simulink model "MainLV1"  (R2024a)
settings: Solver=FixedStepDiscrete  StartTime=0.0  StopTime=Inf  RelTol=1e-3  EnableMultiTasking=on
PreLoadFcn:
  | RTWConfigurationCB('preloadfcn', bdroot);
model workspace (MAT data in the model file):
  fault_count = 0
libraries: canmsglib x11, c280xlib x11, c2837xDlib x5, c2802xlib x5, simulink x4, slpidlib x1
settings Model: ExtModeTrigDuration=8  Creator=Brian  LastModifiedBy=benjaminlevin
settings SolverCC: AutoInsertRateTranBlk=on
settings OptimizationCC: DefaultUnderspecifiedDataType=single  EnhancedBackFolding=on  PassReuseOutputArgsAs=Individual arguments  MaxStackSize=1024  OptimizeBlockOrder=speed  DifferentSizesBufferReuse=on  OptimizationCustomize=off  DenormalBehavior=FlushToZero  EfficientTunableParamExpr=on
settings DebuggingCC: ParameterTunabilityLossMsg=error
settings HardwareCC: ProdBitPerChar=16  ProdBitPerInt=16  ProdBitPerPointer=32  ProdBitPerSizeT=32  ProdBitPerPtrDiffT=32  ProdLargestAtomicInteger=Integer  ProdLargestAtomicFloat=None  ProdWordSize=16  ProdLongLongMode=on  ProdHWDeviceType=Texas Instruments->C2000  HardwareBoardFeatureSet=SoCBlockset
settings ModelReferenceCC: EnableRefExpFcnMdlSchedulingChecks=on  ModelReferenceNumInstancesAllowed=Single
settings SFSimCC: MATLABDynamicMemAlloc=off
settings RTWCC: Description=Embedded Coder  SystemTargetFile=ert.tlc  HardwareBoard=TI Delfino F28379D LaunchPad  TemplateMakefile=ert_default_tmf  Toolchain=Texas Instruments Code Composer Studio (C2000)  CodeProfilingSaveOptions=MetricsOnly  GPUComputeCapability=3.5
settings CodeAppCC: ForceParamTrailComments=on  IgnoreCustomStorageClasses=off  OperatorAnnotations=on  SimulinkDataObjDesc=on  SFDataObjDesc=on  InsertBlockDesc=on
settings ERTTargetCC: CodeReplacementLibrary=TI C28x  ExtModeTransport=4  ExtModeStaticAlloc=on  ExtModeAutomaticAllocSize=off  ExtModeStaticAllocSize=10000  ExtModeMexFile=ext_xcp  ExtModeIntrfLevel=Level2 - Open

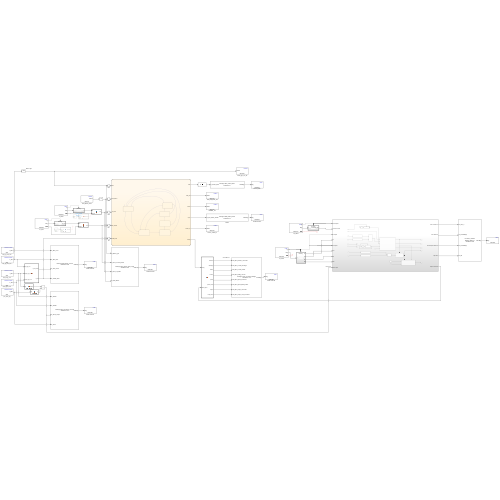
[thumbnail: Simulink's stored preview of the top-level diagram]
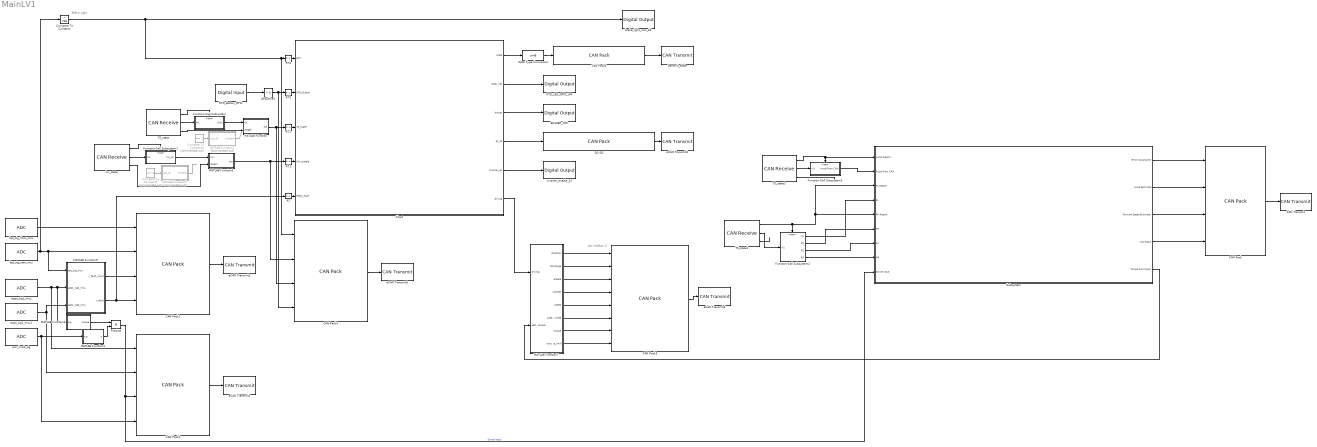
== system MainLV1 ==
  note: Brake Light
  note: can mailbox 3
  BUZZER_105 : c2837xDlib/Digital Output  GPIO_Number=GPIO104~GPIO111  GPIO_Bit0=off  GPIO_BIT0_Toggle=off  GPIO_Bit1=on  GPIO_BIT1_Toggle=off  GPIO_Bit2=off  GPIO_BIT2_Toggle=off  GPIO_Bit3=off  GPIO_BIT3_Toggle=off  GPIO_Bit4=off  GPIO_BIT4_Toggle=off  GPIO_Bit5=off  GPIO_BIT5_Toggle=off  GPIO_Bit6=off  GPIO_BIT6_Toggle=off  GPIO_Bit7=off  GPIO_BIT7_Toggle=off
  CAN Pack : canmsglib/CAN Pack  MsgList=(none)  MsgName=M404_LV  MsgIDType=Standard (11-bit identifier)  MsgIdentifier=404  MsgLength=8  Remote=off  ApplyMinMax=off  BusOutput=off  SignalInfo={ 'LV_COV_V', '32', '8', 'LE', 'unsigned', 'Standard', '0', '0.02', '0', '0', '5.1'; 'LV_FILTERED_A', '16', '16', 'LE', 'unsigned', 'Standard', '0', '5e-05', '0', '0', '3.2767'; 'LV_FILTERED_V', '0', '16', 'LE', 'unsigned', 'Standard', '0', '0.0025', '0', '0', '163.8375'; 'LV_SR', '48', '16', 'LE', 'signed', 'Standard', '0', '0.0001', '0', '-3.2768', '3.2767' }
      settings: LibrarySourceBlock=c2000lib/Target Communication/CAN Pack  DataFormat=manually specified signals
  CAN Pack1 : canmsglib/CAN Pack  MsgList=(none)  MsgName=M402_Brake_Controls  MsgIDType=Standard (11-bit identifier)  MsgIdentifier=402  MsgLength=6  Remote=off  ApplyMinMax=off  BusOutput=off  SignalInfo={'LV_BPT_Front','16','16','LE','unsigned','Standard','0','1','0','-Inf','Inf';'LV_BPT_Rear','0','16','LE','unsigned','Standard','0','1','0','-Inf','Inf';'LV_Fault_Count','40','8','LE','unsigned','Standard','0','1','0','-Inf','Inf';'LV_Pedals_Fault','32','8','LE','signed','Standard','0','1','0','-Inf','Inf'}
      settings: DataFormat=manually specified signals
  CAN Pack2 : canmsglib/CAN Pack  MsgList=(none)  MsgName=M401_Accelerator_Controls  MsgIDType=Standard (11-bit identifier)  MsgIdentifier=401  MsgLength=8  Remote=off  ApplyMinMax=off  BusOutput=off  SignalInfo={'LV_APPS1','0','16','LE','unsigned','Standard','0','1','0','-Inf','Inf';'LV_APPS2','16','16','LE','unsigned','Standard','0','1','0','-Inf','Inf';'LV_Driver_Torque','48','16','LE','signed','Standard','0','0.1','0','-3276.8','3276.7';'LV_Knob','32','16','LE','unsigned','Standard','0','1','0','-Inf','Inf'}
      settings: DataFormat=manually specified signals
  CAN Pack3 : canmsglib/CAN Pack  MsgList=(none)  MsgName=M176_Command_Message  MsgIDType=Standard (11-bit identifier)  MsgIdentifier=176  MsgLength=8  Remote=off  ApplyMinMax=off  BusOutput=off  SignalInfo={'VCU_INV_Direction_Command','32','1','LE','unsigned','Standard','0','1','0','0','1';'VCU_INV_Inverter_Discharge','41','1','LE','unsigned','Standard','0','1','0','0','1';'VCU_INV_Inverter_Enable','40','1','LE','unsigned','Standard','0','1','0','0','1';'VCU_INV_Rolling_Counter','44','4','LE','unsigned','Standard','0','1','0','0','15';'VCU_INV_Speed_Command','16','16','LE','signed','Standard','0','1','0','-32768','32767';'VCU_INV_Speed_Mode_Enable','42','1','LE','unsigned','Standard','0','1','0','0','1';'VCU_INV_Torque_Command','0','16','LE','signed','Standard','0','0.1','0','-3276.8','3276.7';'VCU_INV_Torque_Limit_Command','48','16','LE','signed','Standard','0','0.1','0','-3276.8','3276.7'}
      settings: DataFormat=manually specified signals
  CAN Pack4 : canmsglib/CAN Pack  MsgList=(none)  MsgName=M001_Vehicle_State  MsgIDType=Standard (11-bit identifier)  MsgIdentifier=1  MsgLength=1  Remote=off  ApplyMinMax=off  BusOutput=off  SignalInfo={'LV_Vehicle_State','0','8','LE','signed','Standard','0','1','0','-Inf','Inf'}
      settings: DataFormat=manually specified signals
  CAN Pack5 : canmsglib/CAN Pack  MsgList=(none)  MsgName=M403_Vehicle_State_Inputs  MsgIDType=Standard (11-bit identifier)  MsgIdentifier=403  MsgLength=4  Remote=off  ApplyMinMax=off  BusOutput=off  SignalInfo={'LV_Brake_Light','0','8','LE','unsigned','Standard','0','1','0','-Inf','Inf';'LV_Echo_Inverter_Enable','8','8','LE','signed','Standard','0','1','0','-Inf','Inf';'LV_Echo_TS_State','16','8','LE','signed','Standard','0','1','0','-Inf','Inf';'LV_RTD_Button','24','8','LE','unsigned','Standard','0','1','0','-Inf','Inf'}
      settings: DataFormat=manually specified signals
  CAN Transmit : c280xlib/CAN Transmit  chipFamily=C280x  useModule=CAN_A  mailboxNo=11  messageID=404  messageType=Standard (11-bit identifier)  enableBlockingMode=off  postInterrupt=off  interruptLine=0
  Chart : Stateflow chart  TreatAsAtomicUnit=on  SystemSampleTime=0.01
      settings: RTWSystemCode=Inline  RTWFcnNameOpts=Use subsystem name  RTWFileNameOpts=Use subsystem name  PortSchema="{\"entries\":[{\"content\":{\"sides\":[{\"content\":{\"connectorIds\":[\"In1\",\"In2\",\"In5\",\"In4\",\"In3\"]},\"type\":\"ConnectorPlacement.EquallySpacedRectSide\",\"uuid\":\"e489c846-491e-4e82-9c5f-b669d7c96954\"},{\"content\":{\"connectorIds\":[\"Out1\",\"Out2\",\"Out3\",\"Out4\",\"Out5\",\"Out6\"],\"side\":\"RIGHT\"},\"type\":\"ConnectorPlacement.EquallySpacedRectSide\",\"uuid\":\"cbb46da5-6eb6-44f9-baf3-a24ec6c96225\"},{\"content\":{\"side\":\"TOP\"},\"type\":\"ConnectorPlacement.EquallySpacedRectSide\",\"uuid\":\"c6202e3b-aafb-4b81-a309-4cc98c9bb853\"},{\"content\":{\"side\":\"BOTTOM\"},\"type\":\"ConnectorPlacement.EquallySpacedRectSide\",\"uuid\":\"d6a20d7c-ea9b-4afd-8884-952a45f498ea\"}]},\"type\":\"ConnectorPlacement.EquallySpacedConnector\",\"uuid\":\"7c3bea70-19b9-40c4-b7cb-79b1c3f0d3c0\"}],\"packageUris\":[\"http://schema.mathworks.com/mf0/Connector/R2020b\"],\"version\":\"1.0\"}"
  Compare To Constant : simulink/Logic and Bit Operations/Compare To Constant  relop=>  const=728  OutDataTypeStr=boolean
  Compare To Constant4 : simulink/Logic and Bit Operations/Compare To Constant  Commented=on  relop===  const=1  OutDataTypeStr=boolean
  Compare To Constant5 : simulink/Logic and Bit Operations/Compare To Constant  Commented=on  relop===  const=8  OutDataTypeStr=boolean
  DC-DC : canmsglib/CAN Pack  MsgList=(none)  MsgName=M003_DCDC_Enable  MsgIDType=Standard (11-bit identifier)  MsgIdentifier=3  MsgLength=1  Remote=off  ApplyMinMax=off  BusOutput=off  SignalInfo={'LV_ACC_DCDC_Enable','0','8','LE','signed','Standard','0','1','0','-Inf','Inf'}
      settings: DataFormat=manually specified signals
  Data Type Conversion : DataTypeConversion  OutDataTypeStr=uint8  SaturateOnIntegerOverflow=off  RndMeth=Floor
  Function-Call Subsystem : Subsystem  TreatAsAtomicUnit=on
  Function-Call Subsystem1 : Subsystem  TreatAsAtomicUnit=on
  Function-Call Subsystem2 : Subsystem  TreatAsAtomicUnit=on
  Function-Call Subsystem3 : Subsystem  TreatAsAtomicUnit=on
  IsPositive3 : simulink/Logic and Bit Operations/Compare To Zero  relop=>  OutDataTypeStr=boolean
  MATLAB Function : MATLAB Function  TreatAsAtomicUnit=on
  MATLAB Function1 : MATLAB Function  TreatAsAtomicUnit=on
  MATLAB Function2 : MATLAB Function  Commented=on  TreatAsAtomicUnit=on
  MATLAB Function3 : MATLAB Function  TreatAsAtomicUnit=on
  MATLAB Function4 : MATLAB Function  TreatAsAtomicUnit=on
  MATLAB Function5 : MATLAB Function  Commented=on  TreatAsAtomicUnit=on
  MATLAB Function7 : MATLAB Function  TreatAsAtomicUnit=on
  MATLAB Function9 : MATLAB Function  TreatAsAtomicUnit=on
  Product : Product  OutDataTypeStr=double
  RT{,1..4} (5 alike) : RateTransition  OutPortSampleTime=0.01
  RTD_Button_GPIO : c2837xDlib/Digital Input  GPIO_Number=GPIO32~GPIO39  GPIO_Bit0=on  GPIO_Bit1=off  GPIO_Bit2=off  GPIO_Bit3=off  GPIO_Bit4=off  GPIO_Bit5=off  GPIO_Bit6=off  GPIO_Bit7=off  sampleTime=0.1  dataType=uint8  GPIO_Bit0_Qualification=Sync to SYSCLKOUT  GPIO_Bit1_Qualification=Sync to SYSCLKOUT  GPIO_Bit2_Qualification=Sync to SYSCLKOUT  GPIO_Bit3_Qualification=Sync to SYSCLKOUT  GPIO_Bit4_Qualification=Sync to SYSCLKOUT  GPIO_Bit5_Qualification=Sync to SYSCLKOUT  GPIO_Bit6_Qualification=Sync to SYSCLKOUT  GPIO_Bit7_Qualification=Sync to SYSCLKOUT  Qualification_Period=-1
  RTD_LED_GPIO_104 : c2837xDlib/Digital Output  GPIO_Number=GPIO104~GPIO111  GPIO_Bit0=on  GPIO_BIT0_Toggle=off  GPIO_Bit1=off  GPIO_BIT1_Toggle=off  GPIO_Bit2=off  GPIO_BIT2_Toggle=off  GPIO_Bit3=off  GPIO_BIT3_Toggle=off  GPIO_Bit4=off  GPIO_BIT4_Toggle=off  GPIO_Bit5=off  GPIO_BIT5_Toggle=off  GPIO_Bit6=off  GPIO_BIT6_Toggle=off  GPIO_Bit7=off  GPIO_BIT7_Toggle=off
  Subsystem : Subsystem
  TS_state : c280xlib/CAN Receive  chipFamily=C280x  useModule=CAN_B  mailboxNo=2  messageID=2  messageType=Standard (11-bit identifier)  enableAcceptanceFiltering=off  messageIDMask=0  sampleTime=.25  dataType=CAN_MESSAGE_TYPE  outputAction=Reset all fields to zero  initValue=0  outputMessageID=off  outputMessageLength=on  outputMessageTimeStamp=off  postInterrupt=off  interruptLine=0
  TS_state1 : c280xlib/CAN Receive  chipFamily=C280x  useModule=CAN_B  mailboxNo=9  messageID=51  messageType=Standard (11-bit identifier)  enableAcceptanceFiltering=off  messageIDMask=0  sampleTime=-1  dataType=CAN_MESSAGE_TYPE  outputAction=Reset all fields to zero  initValue=0  outputMessageID=off  outputMessageLength=on  outputMessageTimeStamp=off  postInterrupt=on  interruptLine=0
  TS_state2 : c280xlib/CAN Receive  chipFamily=C280x  useModule=CAN_B  mailboxNo=10  messageID=52  messageType=Standard (11-bit identifier)  enableAcceptanceFiltering=off  messageIDMask=0  sampleTime=-1  dataType=CAN_MESSAGE_TYPE  outputAction=Reset all fields to zero  initValue=0  outputMessageID=off  outputMessageLength=on  outputMessageTimeStamp=off  postInterrupt=on  interruptLine=0
  apps_sig1_mcu : c2802xlib/ADC  blkParamProc=C2000_Type4  ADCModule=A  samplingMode=Single sample mode  ADCResolution=12-bit (Single-ended input)  useSOC1=SOC15  useSOC2=SOC0_SOC1  SOCAcquisitionWindow=60  SOCTriggerSource=Software  SOCInterruptTrigger=No ADCINT  Ts=0.001  dType=uint16  postInterrupt=off  interruptSel=ADCINT1  ADCINTContinuous=on  endma=off  chdma=1  conv1=ADCINA0  conv2=ADCINA0 and ADCINB0  conv1_Type4=ADCIN3  conv2_Type4=ADCIN0 and ADCIN1
  apps_sig2_mcu1 : c2802xlib/ADC  blkParamProc=C2000_Type4  ADCModule=C  samplingMode=Single sample mode  ADCResolution=12-bit (Single-ended input)  useSOC1=SOC10  useSOC2=SOC0_SOC1  SOCAcquisitionWindow=60  SOCTriggerSource=Software  SOCInterruptTrigger=No ADCINT  Ts=0.001  dType=uint16  postInterrupt=off  interruptSel=ADCINT1  ADCINTContinuous=on  endma=off  chdma=1  conv1=ADCINA0  conv2=ADCINA0 and ADCINB0  conv1_Type4=ADCIN2  conv2_Type4=ADCIN0 and ADCIN1
  bpt_sig_front_mcu : c2802xlib/ADC  blkParamProc=C2000_Type4  ADCModule=B  samplingMode=Single sample mode  ADCResolution=12-bit (Single-ended input)  useSOC1=SOC6  useSOC2=SOC0_SOC1  SOCAcquisitionWindow=60  SOCTriggerSource=Software  SOCInterruptTrigger=No ADCINT  Ts=0.001  dType=uint16  postInterrupt=off  interruptSel=ADCINT1  ADCINTContinuous=on  endma=off  chdma=1  conv1=ADCINA0  conv2=ADCINA0 and ADCINB0  conv1_Type4=ADCIN3  conv2_Type4=ADCIN0 and ADCIN1
  bpt_sig_rear_mcu : c2802xlib/ADC  blkParamProc=C2000_Type4  ADCModule=C  samplingMode=Single sample mode  ADCResolution=12-bit (Single-ended input)  useSOC1=SOC6  useSOC2=SOC0_SOC1  SOCAcquisitionWindow=60  SOCTriggerSource=Software  SOCInterruptTrigger=No ADCINT  Ts=0.001  dType=uint16  postInterrupt=off  interruptSel=ADCINT1  ADCINTContinuous=on  endma=off  chdma=1  conv1=ADCINA0  conv2=ADCINA0 and ADCINB0  conv1_Type4=ADCIN3  conv2_Type4=ADCIN0 and ADCIN1
  brake_light_mcu_60 : c2837xDlib/Digital Output  GPIO_Number=GPIO56~GPIO63  GPIO_Bit0=off  GPIO_BIT0_Toggle=off  GPIO_Bit1=off  GPIO_BIT1_Toggle=off  GPIO_Bit2=off  GPIO_BIT2_Toggle=off  GPIO_Bit3=off  GPIO_BIT3_Toggle=off  GPIO_Bit4=on  GPIO_BIT4_Toggle=off  GPIO_Bit5=off  GPIO_BIT5_Toggle=off  GPIO_Bit6=off  GPIO_BIT6_Toggle=off  GPIO_Bit7=off  GPIO_BIT7_Toggle=off
  eCAN Transmit1 : c280xlib/CAN Transmit  chipFamily=C280x  useModule=CAN_B  mailboxNo=6  messageID=401  messageType=Standard (11-bit identifier)  enableBlockingMode=off  postInterrupt=off  interruptLine=0
  eCAN Transmit2 : c280xlib/CAN Transmit  chipFamily=C280x  useModule=CAN_B  mailboxNo=7  messageID=402  messageType=Standard (11-bit identifier)  enableBlockingMode=off  postInterrupt=off  interruptLine=0
  eCAN Transmit3 : c280xlib/CAN Transmit  chipFamily=C280x  useModule=CAN_B  mailboxNo=3  messageID=3  messageType=Standard (11-bit identifier)  enableBlockingMode=off  postInterrupt=off  interruptLine=0
  eCAN Transmit4 : c280xlib/CAN Transmit  chipFamily=C280x  useModule=CAN_B  mailboxNo=4  messageID=192  messageType=Standard (11-bit identifier)  enableBlockingMode=off  postInterrupt=off  interruptLine=0
  eCAN Transmit5 : c280xlib/CAN Transmit  chipFamily=C280x  useModule=CAN_B  mailboxNo=8  messageID=403  messageType=Standard (11-bit identifier)  enableBlockingMode=off  postInterrupt=off  interruptLine=0
  inv_state : c280xlib/CAN Receive  chipFamily=C280x  useModule=CAN_B  mailboxNo=5  messageID=154  messageType=Standard (11-bit identifier)  enableAcceptanceFiltering=off  messageIDMask=0  sampleTime=.25  dataType=CAN_MESSAGE_TYPE  outputAction=Reset all fields to zero  initValue=0  outputMessageID=off  outputMessageLength=on  outputMessageTimeStamp=off  postInterrupt=off  interruptLine=0
  inverter_enable_22 : c2837xDlib/Digital Output  GPIO_Number=GPIO16~GPIO23  GPIO_Bit0=off  GPIO_BIT0_Toggle=off  GPIO_Bit1=off  GPIO_BIT1_Toggle=off  GPIO_Bit2=off  GPIO_BIT2_Toggle=off  GPIO_Bit3=off  GPIO_BIT3_Toggle=off  GPIO_Bit4=off  GPIO_BIT4_Toggle=off  GPIO_Bit5=off  GPIO_BIT5_Toggle=off  GPIO_Bit6=on  GPIO_BIT6_Toggle=off  GPIO_Bit7=off  GPIO_BIT7_Toggle=off
  pwr_knob_sig : c2802xlib/ADC  blkParamProc=C2000_Type4  ADCModule=B  samplingMode=Single sample mode  ADCResolution=12-bit (Single-ended input)  useSOC1=SOC10  useSOC2=SOC0_SOC1  SOCAcquisitionWindow=60  SOCTriggerSource=Software  SOCInterruptTrigger=No ADCINT  Ts=0.001  dType=uint16  postInterrupt=off  interruptSel=ADCINT1  ADCINTContinuous=on  endma=off  chdma=1  conv1=ADCINA0  conv2=ADCINA0 and ADCINB0  conv1_Type4=ADCIN2  conv2_Type4=ADCIN0 and ADCIN1
  transmit_state : c280xlib/CAN Transmit  chipFamily=C280x  useModule=CAN_B  mailboxNo=1  messageID=1  messageType=Standard (11-bit identifier)  enableBlockingMode=off  postInterrupt=off  interruptLine=0
  wires:
  Data Type Conversion/1 -> CAN Pack4/1
  TS_state/2 -> Function-Call Subsystem/1(In1)
  MATLAB Function9/2(r_fault) -> RT/1, CAN Pack1/4
  Function-Call Subsystem/1(Out1) -> MATLAB Function/1(ts)
  TS_state/1 -> Function-Call Subsystem/Trigger
  CAN Pack4/1 -> transmit_state/1
  bpt_sig_rear_mcu/1 -> CAN Pack1/2, MATLAB Function9/1(bpt_sig_mcu), Compare To Constant/1
  apps_sig1_mcu/1 -> CAN Pack2/1, MATLAB Function4/1(sig), MATLAB Function9/2(apps_sig1_mcu)
  apps_sig2_mcu1/1 -> MATLAB Function9/3(apps_sig2_mcu), CAN Pack2/2
  RTD_Button_GPIO/1 -> IsPositive3/1
  CAN Pack1/1 -> eCAN Transmit2/1
  pwr_knob_sig/1 -> CAN Pack2/4, MATLAB Function1/1(sig)
  MATLAB Function1/1(p) -> Product/2
  MATLAB Function4/1(torque) -> Product/1
  DC-DC/1 -> eCAN Transmit3/1
  Chart/1(state) -> Data Type Conversion/1
  CAN Pack3/1 -> eCAN Transmit4/1
  bpt_sig_front_mcu/1 -> CAN Pack1/1
  MATLAB Function9/1(r_fault_count) -> CAN Pack1/3
  CAN Pack2/1 -> eCAN Transmit1/1
  TS_state/3 -> MATLAB Function/2(length)
  Compare To Constant4/1 -> MATLAB Function2/1(can_ok)
  MATLAB Function2/1(timeout) -> ?
  inv_state/1 -> Function-Call Subsystem1/Trigger
  inv_state/2 -> Function-Call Subsystem1/1(In1)
  inv_state/3 -> MATLAB Function3/2(length)
  Compare To Constant5/1 -> MATLAB Function5/1(can_ok)
  Function-Call Subsystem1/1(inv_en) -> MATLAB Function3/1(inv)
  MATLAB Function5/1(timeout) -> ?
  Chart/3(buzzer) -> BUZZER_105/1
  Chart/4(dc_dc) -> DC-DC/1
  Chart/5(inverter_en) -> inverter_enable_22/1
  Chart/6(driving) -> MATLAB Function7/1(driving)
  MATLAB Function7/1(direction) -> CAN Pack3/1
  MATLAB Function7/2(discharge) -> CAN Pack3/2
  MATLAB Function7/3(enable) -> CAN Pack3/3
  MATLAB Function7/5(speed) -> CAN Pack3/5
  MATLAB Function7/4(counter) -> CAN Pack3/4
  MATLAB Function7/6(speed_mode) -> CAN Pack3/6
  MATLAB Function7/7(torque) -> CAN Pack3/7
  MATLAB Function7/8(torque_limit) -> CAN Pack3/8
  Compare To Constant/1 -> brake_light_mcu_60/1, CAN Pack5/1, RT4/1
  Chart/2(ready_led) -> RTD_LED_GPIO_104/1
  CAN Pack5/1 -> eCAN Transmit5/1
  IsPositive3/1 -> CAN Pack5/4, RT3/1
  MATLAB Function/1(out) -> CAN Pack5/3, RT2/1
  MATLAB Function3/1(out) -> CAN Pack5/2, RT1/1
  RT/1 -> Chart/3(Pedal_Fault)
  RT1/1 -> Chart/4(INV_enable)
  RT2/1 -> Chart/5(TS_state)
  RT3/1 -> Chart/2(RTD_Button)
  RT4/1 -> Chart/1(BPT)
  Product/1 -> Subsystem/9(Driver Input), CAN Pack2/3  "Driver Input"
  Subsystem/5(Torque Command) -> MATLAB Function7/2(pedal_torque)
  TS_state1/1 -> Subsystem/3(FL Report), Subsystem/5(FR Report), Function-Call Subsystem2/Trigger
  TS_state1/2 -> Function-Call Subsystem2/1(In1)
  TS_state1/3 -> ?
  TS_state2/2 -> Function-Call Subsystem3/1(In1)
  TS_state2/3 -> ?
  Subsystem/1(Error Covariance) -> CAN Pack/1
  Subsystem/2(Accel Estimate) -> CAN Pack/2
  Subsystem/3(Forward Speed Estimate) -> CAN Pack/3
  Subsystem/4(Slip Ratio) -> CAN Pack/4
  CAN Pack/1 -> CAN Transmit/1
  TS_state2/1 -> Subsystem/1(Accel Report), Function-Call Subsystem3/Trigger
  Function-Call Subsystem2/1(FL) -> Subsystem/4(FL)
  Function-Call Subsystem2/2(FR) -> Subsystem/6(FR)
  Function-Call Subsystem2/3(RL) -> Subsystem/7(RL)
  Function-Call Subsystem2/4(RR) -> Subsystem/8(RR)
  Function-Call Subsystem3/1(Accel from CAN) -> Subsystem/2(Accel from CAN)

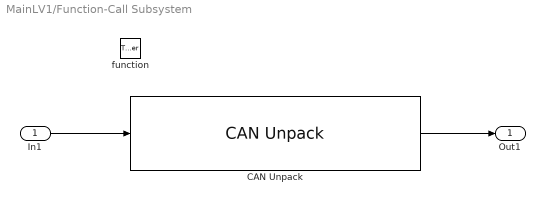
== system MainLV1/Function-Call Subsystem ==
  In1 : Inport
  function : TriggerPort  TriggerType=function-call  VariantControl=(inherit)
  CAN Unpack : canmsglib/CAN Unpack  MsgList=(none)  MsgName=M002_TS_State  MsgIDType=Standard (11-bit identifier)  MsgIdentifier=2  MsgLength=1  SignalInfo={'ACC_TS_State','0','8','LE','signed','Standard','0','1','0','-Inf','Inf'}  IDPort=off  TimestampPort=off  ErrorPort=off  RemotePort=off  LengthPort=off  StatusPort=off  ApplyMinMax=off
  Out1 : Outport  OutDataTypeStr=int8
  wires:
  In1/1 -> CAN Unpack/1
  CAN Unpack/1 -> Out1/1

== system MainLV1/Function-Call Subsystem1 ==
  In1 : Inport
  function : TriggerPort  TriggerType=function-call  VariantControl=(inherit)
  CAN Unpack : canmsglib/CAN Unpack  CANdbFile=C:\Users\lukeh\Documents\FSAE\EV24-Software\CAN\20240129 Gen5 CAN DB.dbc  MsgList=(none)  MsgName=M154_Internal_States  MsgIDType=Standard (11-bit identifier)  MsgIdentifier=154  MsgLength=8  SignalInfo={'INV_BMS_Active','57','1','LE','unsigned','Standard','0','1','0','0','1';'INV_BMS_Torque_Limiting','58','1','LE','unsigned','Standard','0','1','0','0','1';'INV_Burst_Model_Mode','49','1','LE','unsigned','Standard','0','1','0','0','1';'INV_Direction_Command','56','1','LE','unsigned','Standard','0','1','0','0','1';'INV_Inverter_Command_Mode','40','1','LE','unsigned','Standard','0','1','0','0','1';'INV_Inverter_Discharge_State','37','3','LE','unsigned','Standard','0','1','0','0','7';'INV_Inverter_Enable_Lockout','55','1','LE','unsigned','Standard','0','1','0','0','1';'INV_Inverter_Enable_State','48','1','LE','unsigned','Standard','0','1','0','0','1';'INV_Inverter_Run_Mode','32','1','LE','unsigned','Standard','0','1','0','0','1';'INV_Inverter_State','16','8','LE','unsigned','Standard','0','1','0','0','255';'INV_Key_Switch_Start_Status','54','1','LE','unsigned','Standard','0','1','0','0','1';'INV_Limit_Coolant_Derating','62','1','LE','unsigned','Standard','0','1','0','0','1';'INV_Limit_Hot_Spot','60','1','LE','unsigned','Standard','0','1','0','0','1';'INV_Limit_Max_Speed','59','1','LE','unsigned','Standard','0','1','0','0','1';'INV_Limit_Stall_Burst_Model','63','1','LE','unsigned','Standard','0','1','0','0','1';'INV_Low_Speed_Limiting','61','1','LE','unsigned','Standard','0','1','0','0','1';'INV_PWM_Frequency','8','8','LE','unsigned','Standard','0','1','0','0','255';'INV_Relay_1_Status','24','1','LE','unsigned','Standard','0','1','0','0','1';'INV_Relay_2_Status','25','1','LE','unsigned','Standard','0','1','0','0','1';'INV_Relay_3_Status','26','1','LE','unsigned','Standard','0','1','0','0','1';'INV_Relay_4_Status','27','1','LE','unsigned','Standard','0','1','0','0','1';'INV_Relay_5_Status','28','1','LE','unsigned','Standard','0','1','0','0','1';'INV_Relay_6_Status','29','1','LE','unsigned','Standard','0','1','0','0','1';'INV_Rolling_Counter','44','4','LE','unsigned','Standard','0','1','0','0','15';'INV_Self_Sensing_Assist_Enable','33','1','LE','unsigned','Standard','0','1','0','0','1';'INV_VSM_State','0','8','LE','unsigned','Standard','0','1','0','0','15'}  IDPort=off  TimestampPort=off  ErrorPort=off  RemotePort=off  LengthPort=off  StatusPort=off  ApplyMinMax=off
      settings: DataFormat=CANdb specified signals
  inv_en : Outport  OutDataTypeStr=uint8
  wires:
  In1/1 -> CAN Unpack/1
  CAN Unpack/8 -> inv_en/1

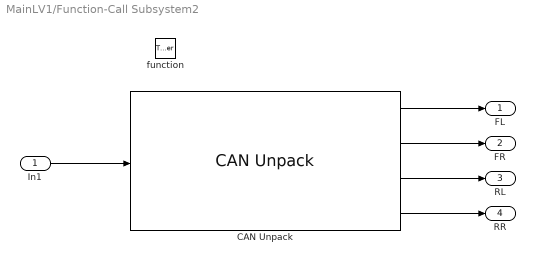
== system MainLV1/Function-Call Subsystem2 ==
  In1 : Inport
  function : TriggerPort  TriggerType=function-call  VariantControl=(inherit)
  CAN Unpack : canmsglib/CAN Unpack  CANdbFile=C:\Users\xudon\OneDrive\Columbia University\FSAE\LV\EV25_CAN.dbc  MsgList=M051_Wheel_Speeds  MsgName=M051_Wheel_Speeds  MsgIDType=Standard (11-bit identifier)  MsgIdentifier=51  MsgLength=8  SignalInfo={ 'SEN_WSS_FL', '0', '16', 'LE', 'unsigned', 'Standard', '0', '0.0025', '0', '0', '163.8375'; 'SEN_WSS_FR', '16', '16', 'LE', 'unsigned', 'Standard', '0', '0.0025', '0', '0', '163.8375'; 'SEN_WSS_RL', '32', '16', 'LE', 'unsigned', 'Standard', '0', '0.0025', '0', '0', '163.8375'; 'SEN_WSS_RR', '48', '16', 'LE', 'unsigned', 'Standard', '0', '0.0025', '0', '0', '163.8375' }  IDPort=off  TimestampPort=off  ErrorPort=off  RemotePort=off  LengthPort=off  StatusPort=off  ApplyMinMax=off
      settings: DataFormat=CANdb specified signals
  FL : Outport  OutDataTypeStr=int8
  FR : Outport  Port=2  OutDataTypeStr=int8
  RL : Outport  Port=3  OutDataTypeStr=int8
  RR : Outport  Port=4  OutDataTypeStr=int8
  wires:
  In1/1 -> CAN Unpack/1
  CAN Unpack/1 -> FL/1
  CAN Unpack/4 -> RR/1
  CAN Unpack/2 -> FR/1
  CAN Unpack/3 -> RL/1

== system MainLV1/Function-Call Subsystem3 ==
  In1 : Inport
  function : TriggerPort  TriggerType=function-call  VariantControl=(inherit)
  CAN Unpack : canmsglib/CAN Unpack  CANdbFile=C:\Users\xudon\OneDrive\Columbia University\FSAE\LV\EV25_CAN.dbc  MsgList=M052_G_Forces  MsgName=M052_G_Forces  MsgIDType=Standard (11-bit identifier)  MsgIdentifier=52  MsgLength=6  SignalInfo={ 'SEN_G_FORCE_X', '0', '16', 'LE', 'unsigned', 'Standard', '0', '5e-05', '0', '0', '3.2767'; 'SEN_G_FORCE_Y', '16', '16', 'LE', 'unsigned', 'Standard', '0', '5e-05', '0', '0', '3.2767'; 'SEN_G_FORCE_Z', '32', '16', 'LE', 'unsigned', 'Standard', '0', '5e-05', '0', '0', '3.2767' }  IDPort=off  TimestampPort=off  ErrorPort=off  RemotePort=off  LengthPort=off  StatusPort=off  ApplyMinMax=off
      settings: DataFormat=CANdb specified signals
  Accel from CAN : Outport  OutDataTypeStr=int8
  wires:
  In1/1 -> CAN Unpack/1
  CAN Unpack/1 -> Accel from CAN/1

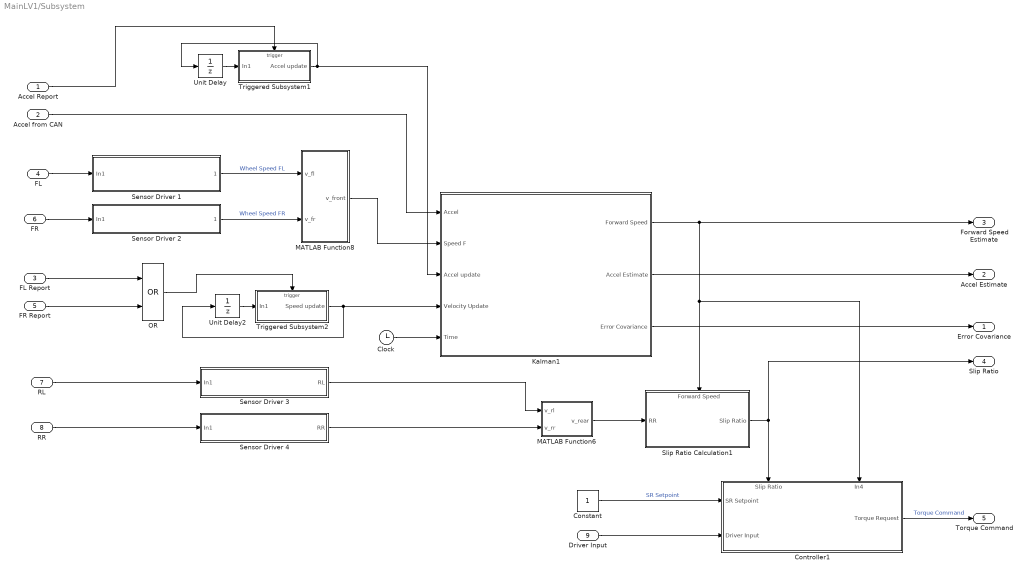
== system MainLV1/Subsystem ==
  Accel Report : Inport
  Accel from CAN : Inport  Port=2
  FL Report : Inport  Port=3
  FL : Inport  Port=4
  FR Report : Inport  Port=5
  FR : Inport  Port=6
  RL : Inport  Port=7
  RR : Inport  Port=8
  Driver Input : Inport  Port=9
  Clock : Clock
  Constant : Constant
  Controller1 : Subsystem
      settings: PortSchema="{\"entries\":[{\"content\":{\"sides\":[{\"content\":{\"connectorIds\":[\"In1\",\"In2\"]},\"type\":\"ConnectorPlacement.EquallySpacedRectSide\",\"uuid\":\"c0b03cac-8500-440b-9ad3-70bdbcbe41b3\"},{\"content\":{\"connectorIds\":[\"Out1\"],\"side\":\"RIGHT\"},\"type\":\"ConnectorPlacement.EquallySpacedRectSide\",\"uuid\":\"4e59df84-775e-4047-ac34-66ccc124485b\"},{\"content\":{\"connectorIds\":[\"In3\",\"In4\"],\"side\":\"TOP\"},\"type\":\"ConnectorPlacement.EquallySpacedRectSide\",\"uuid\":\"12bec3c0-59ce-461e-8d83-22bbad6940ac\"}]},\"type\":\"ConnectorPlacement.EquallySpacedConnector\",\"uuid\":\"2aa18406-4382-4098-896d-4e093aea1de1\"}],\"packageUris\":[\"http://schema.mathworks.com/mf0/Connector/R2020b\"],\"version\":\"1.0\"}"
  Kalman1 : Subsystem
  MATLAB Function6 : MATLAB Function  TreatAsAtomicUnit=on
  MATLAB Function8 : MATLAB Function  TreatAsAtomicUnit=on
  OR : Logic  Operator=OR  IconShape=distinctive  AllPortsSameDT=off  OutDataTypeStr=boolean
  Sensor Driver 1 : Subsystem
  Sensor Driver 2 : Subsystem
  Sensor Driver 3 : Subsystem
  Sensor Driver 4 : Subsystem
  Slip Ratio Calculation1 : Subsystem
      settings: PortSchema="{\"entries\":[{\"content\":{\"sides\":[{\"content\":{\"connectorIds\":[\"In1\"]},\"type\":\"ConnectorPlacement.EquallySpacedRectSide\",\"uuid\":\"061c82cd-7e9c-4a72-b965-43235230dad9\"},{\"content\":{\"connectorIds\":[\"Out1\"],\"side\":\"RIGHT\"},\"type\":\"ConnectorPlacement.EquallySpacedRectSide\",\"uuid\":\"899eaa50-1c30-4f77-9d66-a8daefd9f1e3\"},{\"content\":{\"connectorIds\":[\"In2\"],\"side\":\"TOP\"},\"type\":\"ConnectorPlacement.EquallySpacedRectSide\",\"uuid\":\"89c07a25-5c36-4b16-a58e-7fbb1fd4b8e3\"}]},\"type\":\"ConnectorPlacement.EquallySpacedConnector\",\"uuid\":\"4f00da10-bd17-48bb-8760-fc873e4c20ca\"}],\"packageUris\":[\"http://schema.mathworks.com/mf0/Connector/R2020b\"],\"version\":\"1.0\"}"
  Triggered Subsystem1 : Subsystem  TreatAsAtomicUnit=on
  Triggered Subsystem2 : Subsystem  TreatAsAtomicUnit=on
  Unit Delay : UnitDelay  SampleTime=-1  HasFrameUpgradeWarning=on
  Unit Delay2 : UnitDelay  SampleTime=-1  HasFrameUpgradeWarning=on
  Error Covariance : Outport
  Accel Estimate : Outport  Port=2
  Forward Speed Estimate : Outport  Port=3
  Slip Ratio : Outport  Port=4
  Torque Command : Outport  Port=5
  wires:
  Kalman1/1(Forward Speed) -> Controller1/4(In4), Slip Ratio Calculation1/2(Forward Speed), Forward Speed Estimate/1
  Slip Ratio Calculation1/1(Slip Ratio) -> Controller1/3(Slip Ratio), Slip Ratio/1
  Triggered Subsystem2/1(Speed update) -> Kalman1/4(Velocity Update), Unit Delay2/1
  FR/1 -> Sensor Driver 2/1(In1)
  Sensor Driver 4/1(RR) -> MATLAB Function6/2(v_rr)
  Unit Delay2/1 -> Triggered Subsystem2/1(In1)
  FL Report/1 -> OR/1
  Sensor Driver 2/1(" ") -> MATLAB Function8/2(v_fr)  "Wheel Speed FR"
  MATLAB Function6/1(v_rear) -> Slip Ratio Calculation1/1(RR)
  OR/1 -> Triggered Subsystem2/Trigger
  Triggered Subsystem1/1(Accel update) -> Unit Delay/1, Kalman1/3(Accel update)
  RL/1 -> Sensor Driver 3/1(In1)
  Sensor Driver 1/1(" ") -> MATLAB Function8/1(v_fl)  "Wheel Speed FL"
  Unit Delay/1 -> Triggered Subsystem1/1(In1)
  MATLAB Function8/1(v_front) -> Kalman1/2(Speed F)
  FL/1 -> Sensor Driver 1/1(In1)
  Sensor Driver 3/1(RL) -> MATLAB Function6/1(v_rl)
  Constant/1 -> Controller1/1(SR Setpoint)  "SR Setpoint"
  FR Report/1 -> OR/2
  Controller1/1(Torque Request) -> Torque Command/1  "Torque Command"
  Accel from CAN/1 -> Kalman1/1(Accel)
  Accel Report/1 -> Triggered Subsystem1/Trigger
  RR/1 -> Sensor Driver 4/1(In1)
  Driver Input/1 -> Controller1/2(Driver Input)
  Clock/1 -> Kalman1/5(Time)
  Kalman1/2(Accel Estimate) -> Accel Estimate/1
  Kalman1/3(Error Covariance) -> Error Covariance/1

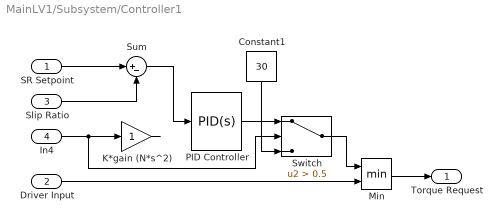
== system MainLV1/Subsystem/Controller1 ==
  SR Setpoint : Inport
  Driver Input : Inport  Port=2
  Slip Ratio : Inport  Port=3
  In4 : Inport  Port=4
  Constant1 : Constant  Value=30
  K*gain (N*s^2) : Gain
  Min : MinMax  Inputs=2
  PID Controller : slpidlib/PID Controller  Controller=PID  Form=Parallel  TimeDomain=Continuous-time  UseExternalTs=off  SampleTime=-1  IntegratorMethod=Forward Euler  FilterMethod=Forward Euler  ControllerParametersSource=internal  P=1  I=1  UseKiTs=off  D=0  UseExternalDerivativeSource=off  N=100  UseFilter=on  TunerSelectOption=Transfer Function Based (PID Tuner App)  InitialConditionSource=internal  InitialConditionForIntegrator=0  InitialConditionForFilter=0  DifferentiatorICPrevScaledInput=0  ExternalReset=none  TrackingMode=off  Kt=1  LimitOutput=on  SatLimitsSource=internal  UpperSaturationLimit=inf  LowerSaturationLimit=-inf  LinearizeAsGain=on  AntiWindupMode=clamping  Kb=1  LimitIntegrator=off  UpperIntegratorSaturationLimit=inf  LowerIntegratorSaturationLimit=-inf  POutMin=[]  POutMax=[]  IOutMin=[]  IOutMax=[]  DOutMin=[]  DOutMax=[]  NOutMin=[]  NOutMax=[]  SumOutMin=[]  SumOutMax=[]  SaturationOutMin=[]  SaturationOutMax=[]  PParamMin=[]  PParamMax=[]  IParamMin=[]  IParamMax=[]  DParamMin=[]  DParamMax=[]  NParamMin=[]  NParamMax=[]  KbParamMin=[]  KbParamMax=[]  KtParamMin=[]  KtParamMax=[]  KbOutMin=[]  KbOutMax=[]  KtOutMin=[]  KtOutMax=[]  IntegratorOutMin=[]  IntegratorOutMax=[]  FilterOutMin=[]  FilterOutMax=[]  SumI1OutMin=[]  SumI1OutMax=[]  SumI2OutMin=[]  SumI2OutMax=[]  SumI3OutMin=[]  SumI3OutMax=[]  SumI4OutMin=[]  SumI4OutMax=[]  SumDOutMin=[]  SumDOutMax=[]  DifferentiatorOutMin=[]  DifferentiatorOutMax=[]  FilterDiffOutCoefMin=[]  FilterDiffOutCoefMax=[]  ReciprocalOutMin=[]  ReciprocalOutMax=[]  SumDenOutMin=[]  SumDenOutMax=[]  SumNumOutMin=[]  SumNumOutMax=[]  DivideOutMin=[]  DivideOutMax=[]  UdiffTsProdOutMin=[]  UdiffTsProdOutMax=[]  NTsProdOutMin=[]  NTsProdOutMax=[]  UintegralTsProdOutMin=[]  UintegralTsProdOutMax=[]  UngainTsProdOutMin=[]  UngainTsProdOutMax=[]  ClampingZeroOutDataTypeStr=Inherit: Inherit via back propagation  ClampingZeroOutMin=[]  ClampingZeroOutMax=[]  FilterDenConstantOutDataTypeStr=Inherit: Inherit via back propagation  FilterDenConstantOutMin=[]  FilterDenConstantOutMax=[]  PCopyOutDataTypeStr=Inherit: Inherit via back propagation  PCopyOutMin=[]  PCopyOutMax=[]  NCopyOutDataTypeStr=Inherit: Inherit via back propagation  NCopyOutMin=[]  NCopyOutMax=[]  IntegratorContinuousStateAttributes=''  IntegratorStateMustResolveToSignalObject=off  IntegratorRTWStateStorageClass=Auto  FilterContinuousStateAttributes=''  FilterStateMustResolveToSignalObject=off  FilterRTWStateStorageClass=Auto  ParallelPVariant=InternalParameters  IdealPVariant=Disabled  IVariant=InternalParameters  DVariant=InternalParameters  IntegratorVariant=Continuous  SatVariant=Enabled  AWVariant=ContClampingParallel  PCopyVariant=Disabled  TRVariant=Disabled  FdbkBlocksVariant=Forward  IdealPFdbkVariant=Disabled  SatFdbkVariant=Disabled  DerivativeFilterVariant=ContFilter  NVariant=InternalParameters  NCopyVariant=Disabled  FilterICVariant=InternalICsFilter  IntegratorICVariant=InternalICs  ExternalResetVariant=Disabled  TRSumVariant=Passthrough  SumFdbkVariant=Disabled  SumVariant=Sum_PID  TsampFilterVariant=InternalTs  TsampNgainVariant=Passthrough  TsampIntegralVariant=Disabled_SignalSpec  ExternalSaturationOutDataTypeStr=Inherit: Same as second input  DerivativeSourceVariant=ErrorSignal
  Sum : Sum  Inputs=|+-
  Switch : Switch  Criteria=u2 > Threshold  Threshold=0.5  SaturateOnIntegerOverflow=off  InputSameDT=off
  Torque Request : Outport
  wires:
  Slip Ratio/1 -> Sum/2
  Sum/1 -> PID Controller/1
  PID Controller/1 -> Switch/1
  Min/1 -> Torque Request/1
  SR Setpoint/1 -> Sum/1
  Driver Input/1 -> Min/2
  K*gain (N*s^2)/1 -> ?
  Constant1/1 -> Switch/3
  In4/1 -> Switch/2, K*gain (N*s^2)/1
  Switch/1 -> Min/1

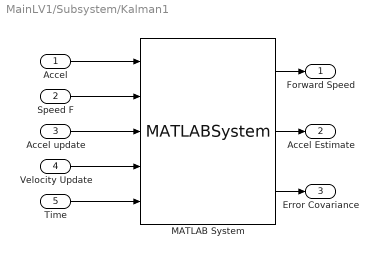
== system MainLV1/Subsystem/Kalman1 ==
  Accel : Inport
  Speed F : Inport  Port=2
  Accel update : Inport  Port=3
  Velocity Update : Inport  Port=4
  Time : Inport  Port=5
  MATLAB System : MATLABSystem  System=Kalman_Filter  qgain=1  SimulateUsing=Code generation
      mask Type: Kalman_Filter
      mask Display:
      | disp('Kalman_Filter');
      | port_label('input',1,'a');
      | port_label('input',2,'v_f');
      | port_label('input',3,'n_a');
      | port_label('input',4,'n_v');
      | port_label('input',5,'t_new');
      | port_label('output',1,'v');
      | port_label('output',2,'a');
      | port_label('output',3,'cov_v');
  Forward Speed : Outport
  Accel Estimate : Outport  Port=2
  Error Covariance : Outport  Port=3
  wires:
  Speed F/1 -> MATLAB System/2
  Accel/1 -> MATLAB System/1
  MATLAB System/1 -> Forward Speed/1
  Accel update/1 -> MATLAB System/3
  Velocity Update/1 -> MATLAB System/4
  Time/1 -> MATLAB System/5
  MATLAB System/2 -> Accel Estimate/1
  MATLAB System/3 -> Error Covariance/1

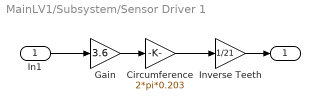
== system MainLV1/Subsystem/Sensor Driver 1 ==
  In1 : Inport
  Circumference : Gain  Gain=2*pi*0.203
  Gain : Gain  Gain=3.6
  Inverse Teeth : Gain  Gain=1/21
  " " : Outport
  wires:
  In1/1 -> Gain/1
  Gain/1 -> Circumference/1
  Circumference/1 -> Inverse Teeth/1
  Inverse Teeth/1 -> " "/1

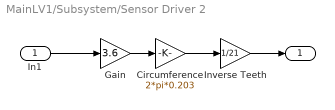
== system MainLV1/Subsystem/Sensor Driver 2 ==
  In1 : Inport
  Circumference : Gain  Gain=2*pi*0.203
  Gain : Gain  Gain=3.6
  Inverse Teeth : Gain  Gain=1/21
  " " : Outport
  wires:
  Circumference/1 -> Inverse Teeth/1
  Inverse Teeth/1 -> " "/1
  In1/1 -> Gain/1
  Gain/1 -> Circumference/1

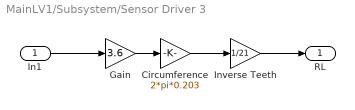
== system MainLV1/Subsystem/Sensor Driver 3 ==
  In1 : Inport
  Circumference : Gain  Gain=2*pi*0.203
  Gain : Gain  Gain=3.6
  Inverse Teeth : Gain  Gain=1/21
  RL : Outport
  wires:
  Circumference/1 -> Inverse Teeth/1
  Inverse Teeth/1 -> RL/1
  In1/1 -> Gain/1
  Gain/1 -> Circumference/1

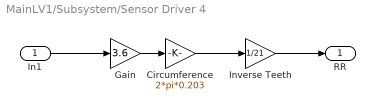
== system MainLV1/Subsystem/Sensor Driver 4 ==
  In1 : Inport
  Circumference : Gain  Gain=2*pi*0.203
  Gain : Gain  Gain=3.6
  Inverse Teeth : Gain  Gain=1/21
  RR : Outport
  wires:
  Circumference/1 -> Inverse Teeth/1
  Inverse Teeth/1 -> RR/1
  In1/1 -> Gain/1
  Gain/1 -> Circumference/1

== system MainLV1/Subsystem/Slip Ratio Calculation1 ==
  RR : Inport
  Forward Speed : Inport  Port=2
  MATLAB Function : MATLAB Function  TreatAsAtomicUnit=on
  Slip Ratio : Outport
  wires:
  Forward Speed/1 -> MATLAB Function/1(fwd_speed)
  RR/1 -> MATLAB Function/2(v_rear)
  MATLAB Function/1(y) -> Slip Ratio/1

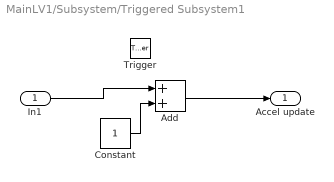
== system MainLV1/Subsystem/Triggered Subsystem1 ==
  In1 : Inport
  Trigger : TriggerPort  VariantControl=(inherit)
  Add : Sum
  Constant : Constant
  Accel update : Outport
  wires:
  In1/1 -> Add/1
  Add/1 -> Accel update/1
  Constant/1 -> Add/2

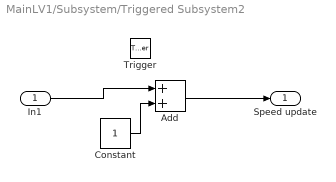
== system MainLV1/Subsystem/Triggered Subsystem2 ==
  In1 : Inport
  Trigger : TriggerPort  VariantControl=(inherit)
  Add : Sum
  Constant : Constant
  Speed update : Outport
  wires:
  In1/1 -> Add/1
  Add/1 -> Speed update/1
  Constant/1 -> Add/2

== matlab function MainLV1/MATLAB Function ==
  data: ts input; out output int8; length input
function out = fcn(ts, length)

% if timeout
%     out = -1; % timeout in TS state CAN signal
persistent timeout;
if isempty(timeout)
    timeout = 0;
end

if length == 0
    timeout = timeout + 1;
else
    timeout = 0;
end

if timeout > 4
    out = int8(-1);
else
    out = int8(ts);
end

== stateflow chart MainLV1/Chart ==
  state State6_Motor_Disabled
    state=6;
    ready_led = 0;
    buzzer = 0;
    inverter_en = 0;
    dc_dc = 0;
    driving = 0;
  state State1_TS_NotReady
    state=1;
    ready_led = 0;
    buzzer = 0;
    inverter_en = 0;
    dc_dc = 0;
    driving = 0;
  state State5_Ready_to_Drive
    state=5;
    ready_led = 0;
    buzzer = 0;
    inverter_en = 1;
    dc_dc = 1;
    driving = 1;
  state State4_Enabling
    state=4;
    ready_led = 0;
    buzzer = 0;
    inverter_en = 1;
    dc_dc = 1;
    driving = 0;
  state State3_Buzzing
    state=3;
    ready_led = 0;
    buzzer = 1;
    inverter_en = 0;
    dc_dc = 1;
    driving = 0;
  state State2_TS_Ready
    state=2;
    ready_led = 1;
    buzzer = 0;
    inverter_en = 0;
    dc_dc = 0;
    driving = 0;
  State3_Buzzing -> State1_TS_NotReady [order 2] : [TS_state ~= 3]
  State5_Ready_to_Drive -> State1_TS_NotReady [order 2] : [TS_state ~= 3]
  State6_Motor_Disabled -> State1_TS_NotReady [order 1] : [TS_state ~= 3]
  (default) -> State1_TS_NotReady
  State4_Enabling -> State6_Motor_Disabled [order 2] : [Pedal_Fault ~= 0]
  State6_Motor_Disabled -> State2_TS_Ready [order 2] : [Pedal_Fault == 0]
  State5_Ready_to_Drive -> State6_Motor_Disabled [order 1] : [Pedal_Fault ~= 0]
  State2_TS_Ready -> State1_TS_NotReady [order 2] : [TS_state ~= 3]
  State1_TS_NotReady -> State2_TS_Ready : [TS_state == 3]
  State5_Ready_to_Drive -> State2_TS_Ready [order 3] : [INV_enable ~= 1]
  State4_Enabling -> State5_Ready_to_Drive [order 1] : [INV_enable == 1]
  State3_Buzzing -> State4_Enabling [order 1] : after(3,sec)
  State2_TS_Ready -> State3_Buzzing [order 1] : [BPT==1&&RTD_Button==1]
  data: BPT input; RTD_Button input; Pedal_Fault input; INV_enable input; TS_state input; state output; ready_led output; buzzer output; dc_dc output; inverter_en output; driving output

== matlab function MainLV1/MATLAB Function2 ==
  data: can_ok input; timeout output
function timeout = ts_chilin(can_ok)

persistent counter;
TS_CAN_COUNT = 3; % 3 samples at 10Hz is a 300ms timeout

% initialize counter
if isempty(counter)
    counter = 0;
end

if can_ok
    counter = 0;
else
    counter = counter + 1;
end

if counter > TS_CAN_COUNT
    timeout = 1;
else
    timeout = 0;
end

== matlab function MainLV1/MATLAB Function3 ==
  data: inv input; out output int8; length input
function out = fcn(inv, length)

% if timeout
%     out = -1; % timeout in TS state CAN signal
persistent timeout;
if isempty(timeout)
    timeout = 0;
end

if length == 0
    timeout = timeout + 1;
else
    timeout = 0;
end

if timeout > 4
    out = int8(-1);
else
    out = int8(inv);
end

== matlab function MainLV1/MATLAB Function4 ==
  data: sig input; torque output
function torque = map_apps1(sig)

APPS_MIN = 1380;
APPS_MAX = 2474;

TORQUE_MIN = 0;
TORQUE_MAX = 140; % max torque in N.m

if sig < APPS_MIN
    torque = TORQUE_MIN;
elseif sig > APPS_MAX
    torque = TORQUE_MAX;
else
    torque = TORQUE_MIN + (TORQUE_MAX - TORQUE_MIN) * (double(sig) - APPS_MIN) / (APPS_MAX - APPS_MIN);
end

== matlab function MainLV1/MATLAB Function5 ==
  data: can_ok input; timeout output
function timeout = inv_chillin(can_ok)

persistent counter;
INV_CAN_COUNT = 3; % 3 samples at 10Hz is a 300ms timeout

% initialize counter
if isempty(counter)
    counter = 0;
end

if can_ok
    counter = 0;
else
    counter = counter + 1;
end

if counter > INV_CAN_COUNT
    timeout = 1;
else
    timeout = 0;
end

== matlab function MainLV1/MATLAB Function7 ==
  data: driving input; pedal_torque input; direction output; discharge output; enable output; counter output; speed output; speed_mode output; torque output; torque_limit output
function [direction, discharge, enable, counter, speed, speed_mode, torque, torque_limit]   = fcn(driving, pedal_torque)

persistent my_counter;
if isempty(my_counter)
    my_counter = 0;
else
    my_counter = mod(my_counter + 1, 16);
end

counter = my_counter;

if driving == 1
    torque = pedal_torque;
    speed = 0;
    direction = 1;
    enable = 1;
    discharge = 0;
    speed_mode = 0;
    torque_limit = 0;
else
    torque = 0;
    speed = 0;
    direction = 0;
    enable = 0;
    discharge = 0;
    speed_mode = 0;
    torque_limit = 0;
end

== matlab function MainLV1/Subsystem/MATLAB Function6 ==
  data: v_rl input; v_rear output; v_rr input
function v_rear = fcn(v_rl,v_rr)
if(v_rl == 0)
    v_rear = v_rr;
else if(v_rr == 0)
    v_rear = v_rl;
else
    v_rear= (v_rl+v_rr)/2;
end
end

== matlab function MainLV1/MATLAB Function9 ==
  data: r_fault_count output; r_fault output; bpt_sig_mcu input; apps_sig1_mcu input; apps_sig2_mcu input
function [r_fault_count, r_fault] = fcn(bpt_sig_mcu, apps_sig1_mcu, apps_sig2_mcu)
%#codegen
%To map voltages / integers:
%Pre step down voltages (from sensors, range 0 to 5 V) * 2/3 -> Post step down voltages (0 to 3.3 V, used by mcu)
%Post step down voltages * (4096 / 3.3) -> uint16 (integer) value of variables
%Note: Some values are tweaked after testing to handle noise. 455 -> 435, 0.1 -> 0.13, etc. All values can and should be optimized from testing, especially from testing on the car

%Current operating range (MCU): 0.32 V to 2.67 V
%Brakes considered pressed: 0.40 V
%typical MCU noise: +- 0.03V

persistent fault_count;
persistent fault;

% initialize persistents
if isempty(fault_count)
    fault_count = 0;
end

if isempty(fault)
    fault = 0;
end

% fault = 0;
apps1_percent_pressed = 0;
apps2_percent_pressed = 0;

% Clear fault case 3 only if APPS less than 5% pressed. 
if (fault == 3)
 if (apps_sig1_mcu < 1000)
        fault = 0;
 end

else 
 % Case 1: Outside operating range.
 if ((apps_sig1_mcu < 800) || (apps_sig2_mcu < 800) || (bpt_sig_mcu < 200) || (apps_sig1_mcu > 4000) || (apps_sig2_mcu > 4000) || (bpt_sig_mcu > 4000))
     fault_count = fault_count + 1;
     if (fault_count > 1000) % corresponds to 1s based on input sampling rate: samples voltage every 1ms (in ADC block, see "Sample time")
         fault = 1;
     else 
         fault = 0;
     end

 apps1_percent_pressed = (double(apps_sig1_mcu) - 1380)/(2474 - 1380); % current travel divided by range of travel
 apps2_percent_pressed = (double(apps_sig2_mcu) - 1008)/(1696 - 1008);

 %Case 2: Both APPs sensors are within operating range but differ by more than 10% for more than 100ms. 
 elseif (abs(apps1_percent_pressed - apps2_percent_pressed) > 0.1)
     fault_count = fault_count + 1;
     if (fault_count > 100) % corresponds to 100ms based on input sampling rate: samples voltage every 1ms (in ADC block, see "Sample time")
         fault = 2;  
     else 
         fault = 0;
     end

%  Case 3: If APPS is more than 25% pressed and brakes are pressed.
  elseif (((apps_sig1_mcu > 1700)) && (bpt_sig_mcu > 500))
b         fault = 3;
        
 %No faults    
 else
     fault_count = 0;
     fault = 0;
 end 
end

r_fault_count = fault_count;
r_fault = fault;

== matlab function MainLV1/Subsystem/MATLAB Function8 ==
  data: v_fl input; v_front output; v_fr input
function v_front = fcn(v_fl,v_fr)

if(v_fl == 0)
    v_front = v_fr;
else if(v_fr == 0)
    v_front = v_rl;
else
    v_front= (v_fl+v_fr)/2;
end
end

== matlab function MainLV1/Subsystem/Slip Ratio Calculation1/MATLAB Function ==
  data: fwd_speed input; y output; v_rear input
function y = fcn(fwd_speed,v_rear)

y = (v_rear - fwd_speed)/(max([fwd_speed,0.1]));

== matlab function MainLV1/MATLAB Function1 ==
  data: sig input; p output
function p = map_knob(sig)

KNOB_MIN = 0;
KNOB_MAX = 4095;

P_MIN = 0;
P_MAX = 1;

if sig < KNOB_MIN
    p = P_MIN;
elseif sig > KNOB_MAX
    p = P_MAX;
else
    p = P_MIN + (P_MAX - P_MIN) * (double(sig) - KNOB_MIN) / (KNOB_MAX - KNOB_MIN);
end
